simulink model "Project_Three_1s_Pattern"  (R2023b)
settings: Solver=VariableStepAuto  StartTime=0.0  StopTime=1  RelTol=1e-3
settings Model: Creator=chand  LastModifiedBy=chand

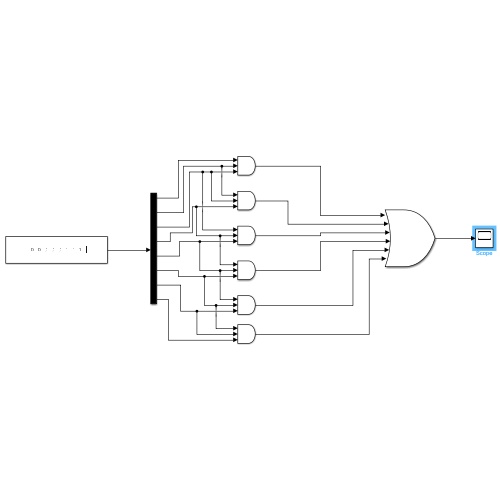
[thumbnail: Simulink's stored preview of the top-level diagram]
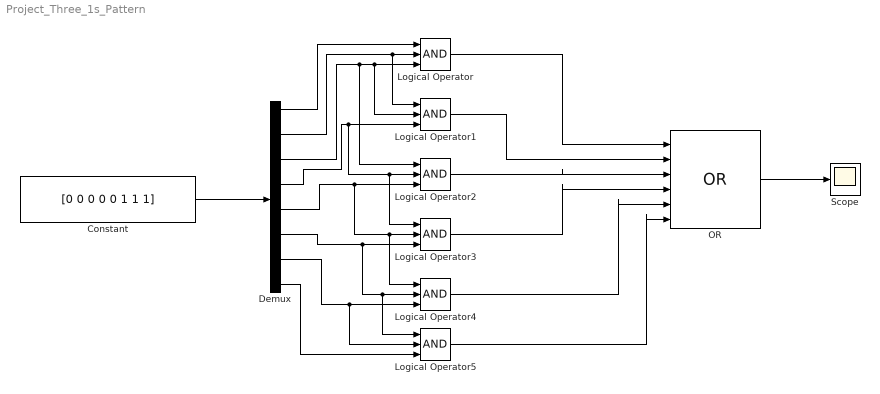
== system Project_Three_1s_Pattern ==
  Constant : Constant  Value=[0 0 0 0 0 1 1 1]
  Demux : Demux  Outputs=8
  Logical Operator{,1..5} (6 alike) : Logic  Inputs=3  IconShape=distinctive  AllPortsSameDT=off  OutDataTypeStr=boolean
  OR : Logic  Operator=OR  Inputs=6  IconShape=distinctive  AllPortsSameDT=off  OutDataTypeStr=boolean
  Scope : Scope
  wires:
  Demux/1 -> Logical Operator/1
  Demux/2 -> Logical Operator1/1, Logical Operator/2
  Demux/3 -> Logical Operator2/1, Logical Operator1/2, Logical Operator/3
  Demux/4 -> Logical Operator3/1, Logical Operator2/2, Logical Operator1/3
  Demux/5 -> Logical Operator4/1, Logical Operator3/2, Logical Operator2/3
  Demux/7 -> Logical Operator5/2, Logical Operator4/3
  Demux/8 -> Logical Operator5/3
  Demux/6 -> Logical Operator5/1, Logical Operator4/2, Logical Operator3/3
  Logical Operator/1 -> OR/1
  Logical Operator1/1 -> OR/2
  Logical Operator2/1 -> OR/3
  Logical Operator3/1 -> OR/4
  Logical Operator4/1 -> OR/5
  Logical Operator5/1 -> OR/6
  OR/1 -> Scope/1
  Constant/1 -> Demux/1
